simulink model "exampleSimulation"  (R2018b)
settings: Solver=ode23tb  StartTime=0.0  StopTime=10.0  RelTol=1e-3
libraries: powerlib x4, powerlib_meascontrol x2, microgridLibrary x1
settings Model: Creator=jlesage  LastModifiedBy=jlesage

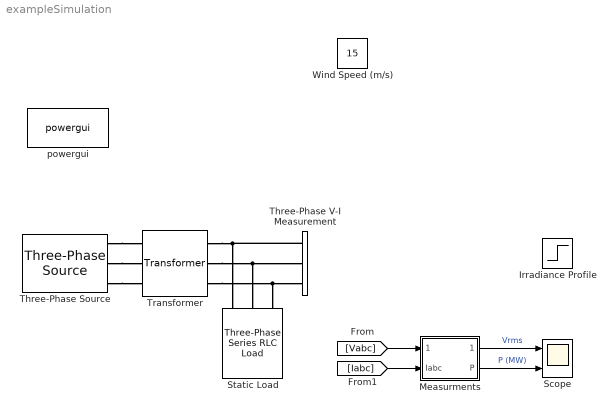
== system exampleSimulation ==
  Irradiance Profile : Step  Time=5  Before=500e3  After=250e3  SampleTime=0
  Measurments : Subsystem
  Scope : Scope  NumInputPorts=2
  Static Load : powerlib/Elements/Three-Phase Series RLC Load  LConnTagsString=A|B|C  Configuration=Y (grounded)  NominalVoltage=5000  Vabc=[1e3 1e3 1e3]  Vabcp=[1e3 1e3 1e3]  NominalFrequency=60  UnbalancedPower=off  ActivePower=100e3  InductivePower=0  CapacitivePower=0  Pabc=[10e3 9e3 11e3]  QLabc=[100 90 110]  QCabc=[100 90 110]  Pabcp=[10e3 9e3 11e3]  QLabcp=[100 90 110]  QCabcp=[100 90 110]  Measurements=None  LoadType=constant Z
      settings: SourceProductName=Simscape Electrical
  Three-Phase V-I Measurement : powerlib/Measurements/Three-Phase V-I Measurement  VoltageMeasurement=phase-to-ground  SetLabelV=on  LabelV=Vabc  Vpu=off  VpuLL=off  CurrentMeasurement=yes  SetLabelI=on  LabelI=Iabc  Ipu=off  Pbase=100e6  Vbase=500e3  OutputType=Complex  PhasorSimulation=on  PSBequivalent=0
  Three-Phase Source : powerlib/Electrical Sources/Three-Phase Source  InternalConnection=Yg  VoltagePhases=off  Voltage=25e3  PhaseAngle=0  Voltage_phases=[25e3 25e3 25e3]/sqrt(3)  PhaseAngles_phases=[0 -120 +120]  Frequency=60  NonIdealSource=on  SpecifyImpedance=off  Resistance=0.8929  Inductance=16.58e-3  ShortCircuitLevel=100e6  BaseVoltage=25e3  XRratio=7  BusType=swing  Pref=10e3  Qref=0  Prefabc=[10e3, 10e3, 10e3]  Qrefabc=[0, 0, 0]  Qmin=-inf  Qmax=inf
  Transformer : microgridLibrary/Transformer  kS=225  Freq=60  Vp=25e3  Vs=5000  Zperc=5.18  Ratio=2.5
  Wind Speed (m/s) : Constant  Value=15
  powergui : powerlib/powergui  Priority=1  SimulationMode=Phasor  SampleTime=50e-6  frequency=60  Iterations=50  frequencyindice=60  Pbase=100e6  ErrMax=1e-4  UnitsV=kV  UnitsW=MW  buscounter=0  FunctionMessages=off  echomessages=off  EnableUseOfTLC=off  CurrentSourceSwitches=off  DisableSnubberDevices=off  DisableRonSwitches=off  DisableVfSwitches=off  DisplayEquations=off  SolverType=Tustin/Backward Euler (TBE)  Interpol=off  ExternalGateDelay=off  methode=off  Ts=100  x0status=blocks  SPID=on  SwTol=0  HookPort=off  RestoreLinks=warning  ResistiveCurrentMeasurement=off  Frange=[0:2:500]  Ylog=off  Xlog=on  ShowGrid=off  save=off  variable=ZData  structure=0  ZoomFFT=off  StartTime=0.0  cycles=1  DisplayStyle=1  fundamental=60  FreqAxis=off  MaxFrequency=1000  frequencyindicesteady=1  RmsSteady=1  display=off
  wires:
  [Vabc] -> Measurments/1(Vabc)
  [Iabc] -> Measurments/2(Iabc)
  Measurments/1(Vrms) -> Scope/1  "Vrms"
  Measurments/2(P) -> Scope/2  "P (MW)"
  connections:
  Three-Phase Source/RConn1 -- Transformer/LConn1
  Three-Phase Source/RConn2 -- Transformer/LConn2
  Three-Phase Source/RConn3 -- Transformer/LConn3
  Transformer/RConn1 -- Three-Phase V-I Measurement/RConn1 -- Static Load/LConn1
  Transformer/RConn2 -- Three-Phase V-I Measurement/RConn2 -- Static Load/LConn2
  Transformer/RConn3 -- Static Load/LConn3 -- Three-Phase V-I Measurement/RConn3

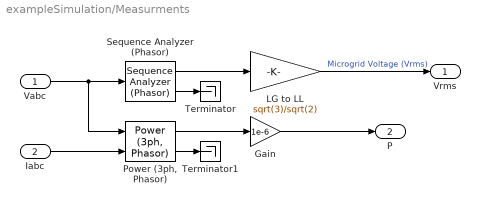
== system exampleSimulation/Measurments ==
  Vabc : Inport
  Iabc : Inport  Port=2
  Gain : Gain  Gain=1e-6
  LG to LL : Gain  Gain=sqrt(3)/sqrt(2)
  "Power (3ph, Phasor)" : powerlib_meascontrol/Measurements/Power (3ph, Phasor)
      settings: SourceProductName=Simscape Power Systems  SourceProductBaseCode=PS
  Sequence Analyzer (Phasor) : powerlib_meascontrol/Measurements/Sequence Analyzer (Phasor)  seq=Positive
      settings: SourceProductName=Simscape Power Systems  SourceProductBaseCode=PS
  Terminator : Terminator
  Terminator1 : Terminator
  Vrms : Outport
  P : Outport  Port=2
  wires:
  Sequence Analyzer (Phasor)/1 -> LG to LL/1
  Sequence Analyzer (Phasor)/2 -> Terminator/1
  LG to LL/1 -> Vrms/1  "Microgrid Voltage (Vrms)"
  Iabc/1 -> "Power (3ph, Phasor)"/2
  Vabc/1 -> "Power (3ph, Phasor)"/1, Sequence Analyzer (Phasor)/1
  "Power (3ph, Phasor)"/2 -> Terminator1/1
  "Power (3ph, Phasor)"/1 -> Gain/1
  Gain/1 -> P/1
